simulink model "Power_split_controller_Bulk_Carrier"  (R2021b)
settings: Solver=VariableStepAuto  StartTime=0.0  StopTime=8210  RelTol=1
undefined symbols (not defined in the file): ISOC, ISOC_bc, Pd_BC, Pl_bc, Pu_bc, QC, QC_bc, R0_bc, SOC_L, V0, V0_bc
libraries: simulink x1
settings Model: Creator=bldha  LastModifiedBy=bldha
settings SolverCC: ZeroCrossAlgorithm=Adaptive
settings DebuggingCC: IgnoredZcDiagnostic=none

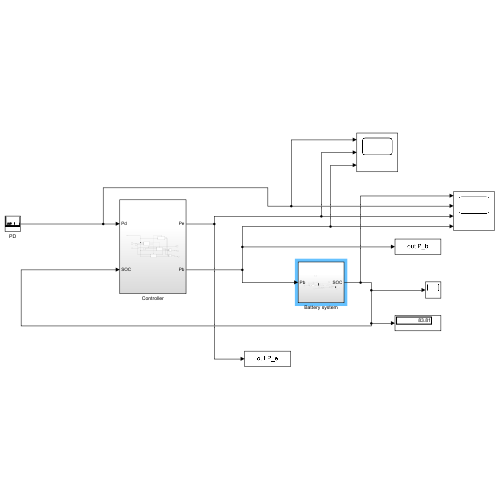
[thumbnail: Simulink's stored preview of the top-level diagram]
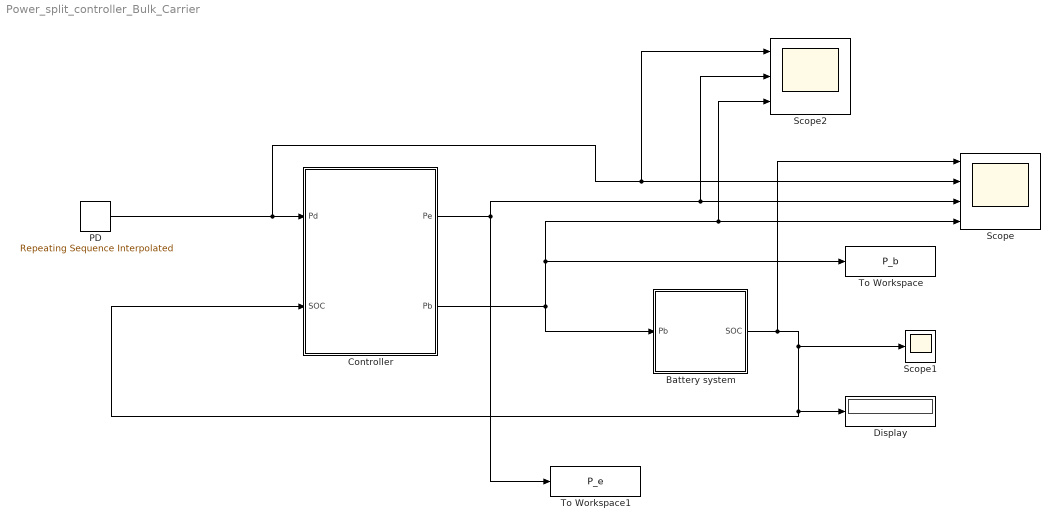
== system Power_split_controller_Bulk_Carrier ==
  Battery system : Subsystem
  Controller : Subsystem
  Display : Display
  PD : simulink/Sources/Repeating Sequence Interpolated  OutValues=[Pd_BC.pow]  TimeValues=[Pd_BC.time]  LookUpMeth=Interpolation-Use End Values  tsamp=0.1  OutMin=[]  OutMax=[]  OutDataTypeStr=double  OutputDataTypeScalingMode=double  OutDataType=fixdt(0,8)  OutScaling=2^-10
  Scope : Scope  NumInputPorts=4
  Scope1 : Scope
  Scope2 : Scope  NumInputPorts=3
  To Workspace : ToWorkspace  VariableName=P_b  SampleTime=-1
  To Workspace1 : ToWorkspace  VariableName=P_e  SampleTime=-1
  wires:
  Battery system/1(SOC) -> Scope/1, Display/1, Controller/2(SOC), Scope1/1
  Controller/1(Pe) -> To Workspace1/1, Scope2/2, Scope/3
  PD/1 -> Controller/1(Pd), Scope2/1, Scope/2
  Controller/2(Pb) -> To Workspace/1, Scope2/3, Scope/4, Battery system/1(Pb)

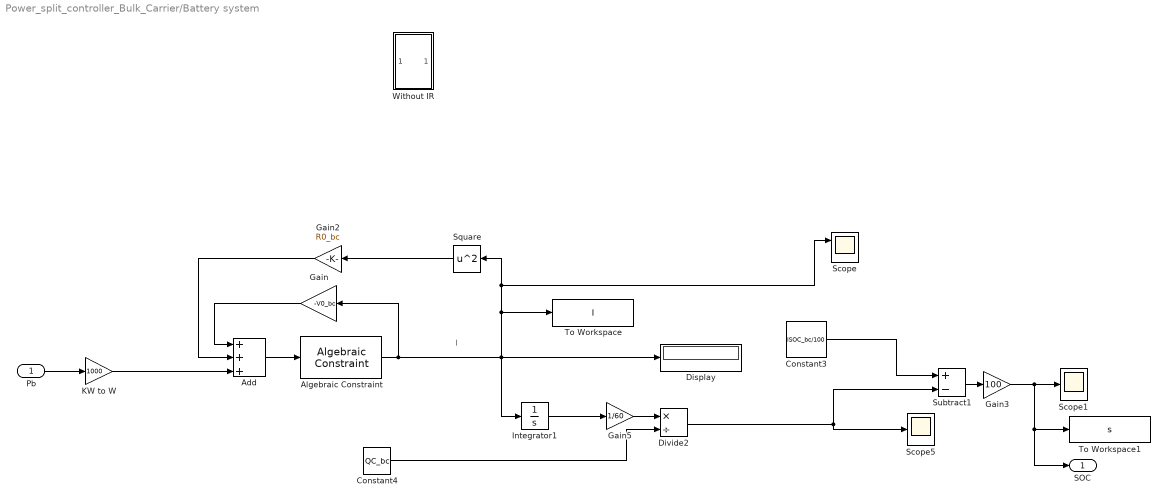
== system Power_split_controller_Bulk_Carrier/Battery system ==
  note: I
  Pb : Inport
  Add : Sum  Inputs=+++
  Algebraic Constraint : AlgebraicConstraint  InitialGuess=-999999999999
  Constant3 : Constant  Value=ISOC_bc/100
  Constant4 : Constant  Value=QC_bc
  Display : Display
  Divide2 : Product  Inputs=*/
  Gain : Gain  Gain=-V0_bc
  Gain2 : Gain  Gain=R0_bc
  Gain3 : Gain  Gain=100
  Gain5 : Gain  Gain=1/60
  Integrator1 : Integrator
  KW to W : Gain  Gain=1000
  Scope : Scope  NumInputPorts=2
  Scope1 : Scope
  Scope5 : Scope
  Square : Math  Operator=square  SaturateOnIntegerOverflow=on
  Subtract1 : Sum  Inputs=+-
  To Workspace : ToWorkspace  VariableName=I  SaveFormat=Structure With Time  SampleTime=-1
  To Workspace1 : ToWorkspace  VariableName=s  SaveFormat=Structure With Time  SampleTime=-1
  Without IR : Subsystem
  SOC : Outport
  wires:
  KW to W/1 -> Add/3
  Gain/1 -> Add/1
  Add/1 -> Algebraic Constraint/1
  Square/1 -> Gain2/1
  Gain2/1 -> Add/2
  Pb/1 -> KW to W/1
  Divide2/1 -> Subtract1/2, Scope5/1
  Constant3/1 -> Subtract1/1
  Subtract1/1 -> Gain3/1
  Gain3/1 -> To Workspace1/1, SOC/1, Scope1/1
  Constant4/1 -> Divide2/2
  Algebraic Constraint/1 -> Gain/1, Square/1, Scope/1, To Workspace/1, Display/1, Integrator1/1
  Gain5/1 -> Divide2/1
  Integrator1/1 -> Gain5/1

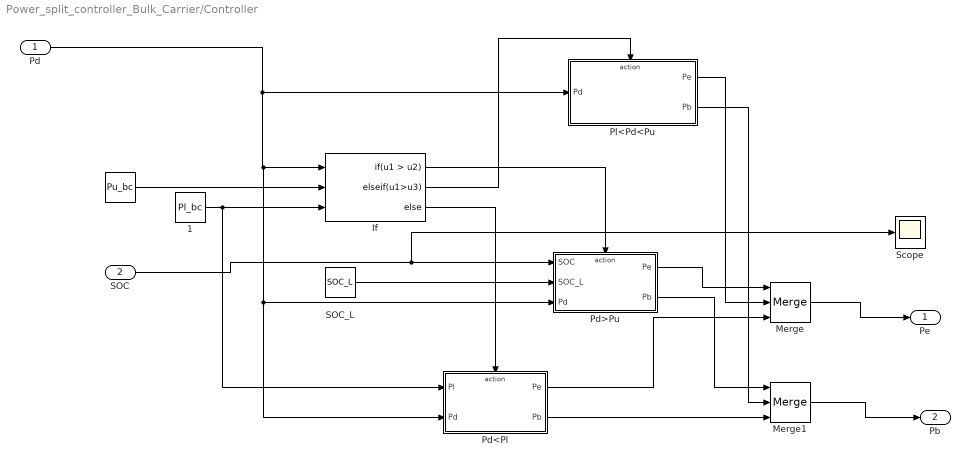
== system Power_split_controller_Bulk_Carrier/Controller ==
  Pd : Inport
  SOC : Inport  Port=2
  "   " : Constant  Value=Pu_bc
  "   1" : Constant  Value=Pl_bc
  If : If  NumInputs=3  IfExpression=u1 > u2  ElseIfExpressions=u1>u3
  Merge : Merge  Inputs=3
  Merge1 : Merge  Inputs=3
  Pd<Pl : Subsystem  TreatAsAtomicUnit=on
  Pd>Pu : Subsystem  TreatAsAtomicUnit=on
  Pl<Pd<Pu : Subsystem  TreatAsAtomicUnit=on
  SOC_L : Constant  Value=SOC_L
  Scope : Scope
  Pe : Outport
  Pb : Outport  Port=2
  wires:
  SOC/1 -> Scope/1, Pd>Pu/1(SOC)
  Merge1/1 -> Pb/1
  Pd/1 -> Pd>Pu/3(Pd), Pd<Pl/2(Pd), If/1, Pl<Pd<Pu/1(Pd)
  Merge/1 -> Pe/1
  "   "/1 -> If/2
  Pl<Pd<Pu/1(Pe) -> Merge/2
  Pd>Pu/2(Pb) -> Merge1/1
  Pd>Pu/1(Pe) -> Merge/1
  Pd<Pl/1(Pe) -> Merge/3
  Pd<Pl/2(Pb) -> Merge1/3
  Pl<Pd<Pu/2(Pb) -> Merge1/2
  If/3 -> Pd<Pl/Action
  "   1"/1 -> Pd<Pl/1(Pl), If/3
  If/2 -> Pl<Pd<Pu/Action
  SOC_L/1 -> Pd>Pu/2(SOC_L)
  If/1 -> Pd>Pu/Action

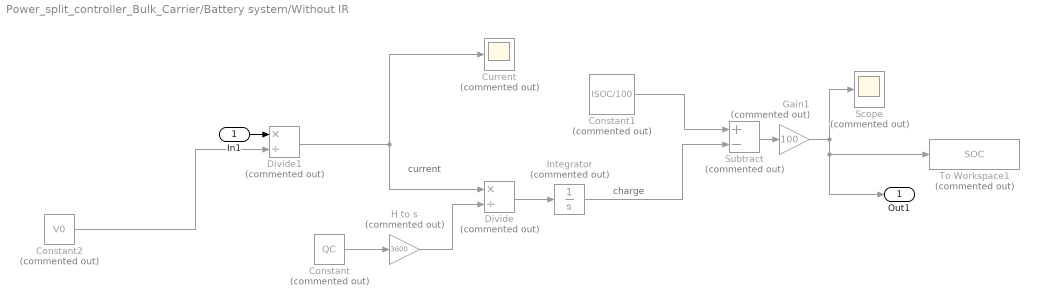
== system Power_split_controller_Bulk_Carrier/Battery system/Without IR ==
  note: current
  note: charge
  In1 : Inport
  Constant : Constant  Commented=on  Value=QC
  Constant1 : Constant  Commented=on  Value=ISOC/100
  Constant2 : Constant  Commented=on  Value=V0
  Current : Scope  Commented=on
  Divide : Product  Commented=on  Inputs=*/
  Divide1 : Product  Commented=on  Inputs=*/
  Gain1 : Gain  Commented=on  Gain=100
  H to s : Gain  Commented=on  Gain=3600
  Integrator : Integrator  Commented=on
  Scope : Scope  Commented=on
  Subtract : Sum  Commented=on  Inputs=+-
  To Workspace1 : ToWorkspace  Commented=on  VariableName=SOC  SampleTime=-1
  Out1 : Outport
  wires:
  Subtract/1 -> Gain1/1
  Constant2/1 -> Divide1/2
  Gain1/1 -> Out1/1, To Workspace1/1, Scope/1
  Constant/1 -> H to s/1
  Divide1/1 -> Divide/1, Current/1
  H to s/1 -> Divide/2
  Divide/1 -> Integrator/1
  Integrator/1 -> Subtract/2
  Constant1/1 -> Subtract/1
  In1/1 -> Divide1/1

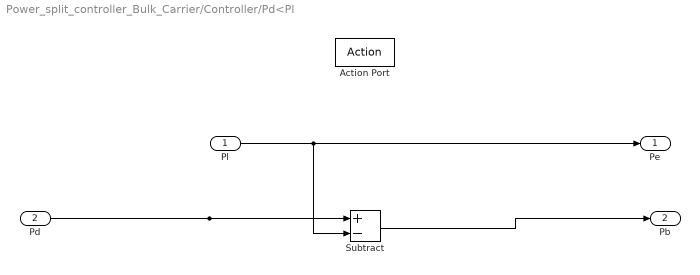
== system Power_split_controller_Bulk_Carrier/Controller/Pd<Pl ==
  Pl : Inport
  Pd : Inport  Port=2
  Action Port : ActionPort  ActionPortLabel=else
  Subtract : Sum  Inputs=+-
  Pe : Outport
  Pb : Outport  Port=2
  wires:
  Pl/1 -> Subtract/2, Pe/1
  Pd/1 -> Subtract/1
  Subtract/1 -> Pb/1

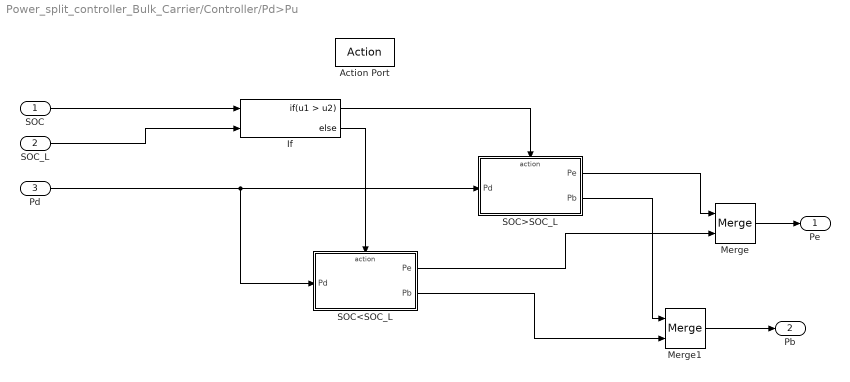
== system Power_split_controller_Bulk_Carrier/Controller/Pd>Pu ==
  SOC : Inport
  SOC_L : Inport  Port=2
  Pd : Inport  Port=3
  Action Port : ActionPort  ActionPortLabel=if(u1 > u2)
  If : If  NumInputs=2  IfExpression=u1 > u2
  Merge : Merge
  Merge1 : Merge
  SOC<SOC_L : Subsystem  TreatAsAtomicUnit=on
  SOC>SOC_L : Subsystem  TreatAsAtomicUnit=on
  Pe : Outport
  Pb : Outport  Port=2
  wires:
  SOC/1 -> If/1
  SOC_L/1 -> If/2
  If/1 -> SOC>SOC_L/Action
  If/2 -> SOC<SOC_L/Action
  SOC>SOC_L/1(Pe) -> Merge/1
  SOC<SOC_L/1(Pe) -> Merge/2
  Merge/1 -> Pe/1
  SOC>SOC_L/2(Pb) -> Merge1/1
  SOC<SOC_L/2(Pb) -> Merge1/2
  Merge1/1 -> Pb/1
  Pd/1 -> SOC<SOC_L/1(Pd), SOC>SOC_L/1(Pd)

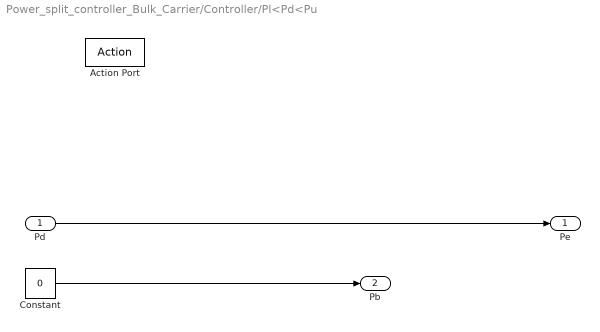
== system Power_split_controller_Bulk_Carrier/Controller/Pl<Pd<Pu ==
  Pd : Inport
  Action Port : ActionPort  ActionPortLabel=elseif(u1>u3)
  Constant : Constant  Value=0
  Pe : Outport
  Pb : Outport  Port=2
  wires:
  Pd/1 -> Pe/1
  Constant/1 -> Pb/1

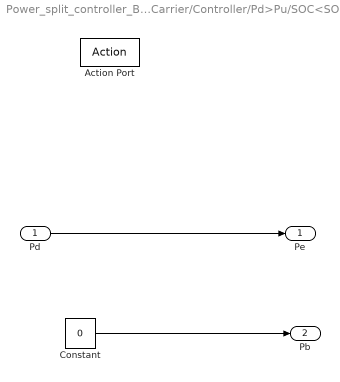
== system Power_split_controller_Bulk_Carrier/Controller/Pd>Pu/SOC<SOC_L ==
  Pd : Inport
  Action Port : ActionPort  ActionPortLabel=else
  Constant : Constant  Value=0
  Pe : Outport
  Pb : Outport  Port=2
  wires:
  Constant/1 -> Pb/1
  Pd/1 -> Pe/1

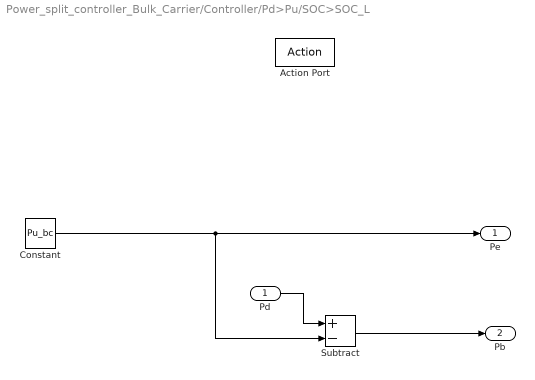
== system Power_split_controller_Bulk_Carrier/Controller/Pd>Pu/SOC>SOC_L ==
  Pd : Inport
  Action Port : ActionPort  ActionPortLabel=if(u1 > u2)
  Constant : Constant  Value=Pu_bc
  Subtract : Sum  Inputs=+-
  Pe : Outport
  Pb : Outport  Port=2
  wires:
  Constant/1 -> Subtract/2, Pe/1
  Pd/1 -> Subtract/1
  Subtract/1 -> Pb/1
